simulink library "INT_SSpMon_Co"  (R2016b)
settings: Solver=VariableStepAuto  StartTime=0.0  StopTime=10.0  RelTol=1e-3
settings Model: Creator=Administrator  LastModifiedBy=Administrator

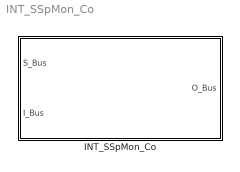
== system INT_SSpMon_Co ==
  INT_SSpMon_Co : Subsystem

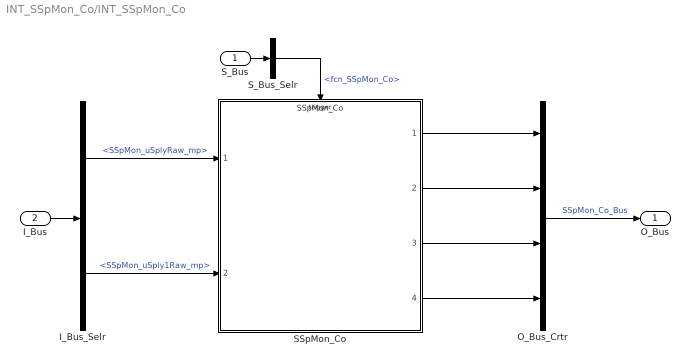
== system INT_SSpMon_Co/INT_SSpMon_Co ==
  S_Bus : Inport
  I_Bus : Inport  Port=2
  I_Bus_Selr : BusSelector  OutputSignals=SSpMon_uSplyRaw_mp,SSpMon_uSply1Raw_mp
  O_Bus_Crtr : BusCreator  Inputs=4
  SSpMon_Co : ModelReference  ModelNameDialog=SSpMon_Co  SimulationMode=Normal  ModelReferenceVersion=1.8  TriggerPortName=function  TriggerPortTriggerType=function-call  TriggerPortStatesWhenEnabling=held
  S_Bus_Selr : BusSelector  OutputSignals=fcn_SSpMon_Co
  O_Bus : Outport
  wires:
  S_Bus_Selr/1 -> SSpMon_Co/Trigger  "<fcn_SSpMon_Co>"
  S_Bus/1 -> S_Bus_Selr/1
  I_Bus/1 -> I_Bus_Selr/1
  I_Bus_Selr/1 -> SSpMon_Co/1  "<SSpMon_uSplyRaw_mp>"
  I_Bus_Selr/2 -> SSpMon_Co/2  "<SSpMon_uSply1Raw_mp>"
  O_Bus_Crtr/1 -> O_Bus/1  "SSpMon_Co_Bus"
  SSpMon_Co/1 -> O_Bus_Crtr/1
  SSpMon_Co/2 -> O_Bus_Crtr/2
  SSpMon_Co/3 -> O_Bus_Crtr/3
  SSpMon_Co/4 -> O_Bus_Crtr/4
